simulink model "Diagram"  (R2015b)
settings: Solver=VariableStepAuto  StartTime=0.0  StopTime=0.15  RelTol=1e-3
undefined symbols (not defined in the file): K2, L2, sysog
libraries: simulink x1
settings Model: Creator=zap  LastModifiedBy=zap

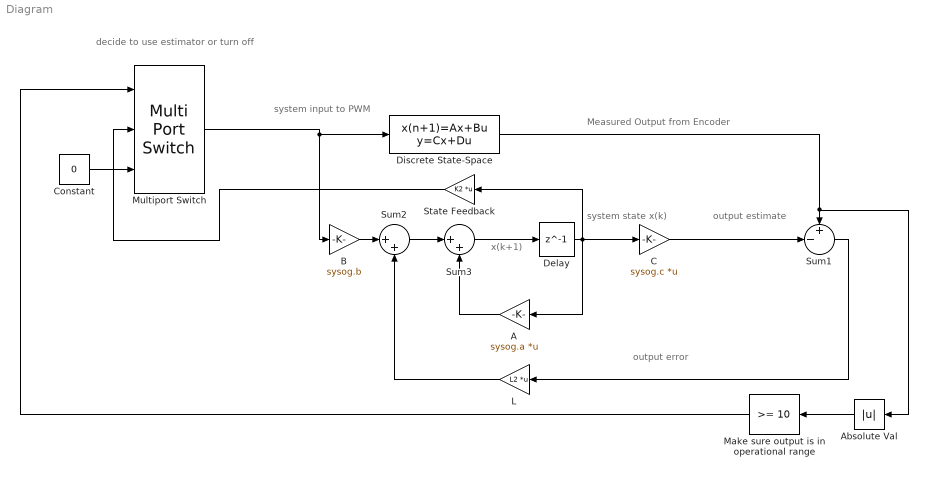
== system Diagram ==
  note: decide to use estimator or turn off
  note: system input to PWM
  note: x(k+1)
  note: system
      | state x(k)
  note: output error
  note: Measured Output from Encoder
  note: output estimate
  A : Gain  Gain=sysog.a  Multiplication=Matrix(K*u)
  Absolute Val : Abs
  B : Gain  Gain=sysog.b
  C : Gain  Gain=sysog.c  Multiplication=Matrix(K*u)
  Constant : Constant  Value=0
  Delay : Delay  DelayLength=1  InitialCondition=0
  Discrete State-Space : DiscreteStateSpace  A=sysog.a  B=sysog.b  C=sysog.c  D=sysog.d  SampleTime=10^-4
  L : Gain  Gain=L2  Multiplication=Matrix(K*u)
  Make sure output is in operational range : simulink/Logic and Bit Operations/Compare To Constant  relop=>=  const=10  OutDataTypeStr=boolean
  Multiport Switch : MultiPortSwitch  Inputs=2
  State Feedback : Gain  Gain=K2  Multiplication=Matrix(K*u)
  Sum1 : Sum  Inputs=+-|
  Sum2 : Sum  Inputs=|++
  Sum3 : Sum  Inputs=|++
  wires:
  Discrete State-Space/1 -> Absolute Val/1, Sum1/1
  Multiport Switch/1 -> B/1, Discrete State-Space/1
  B/1 -> Sum2/1
  Sum2/1 -> Sum3/1
  Sum3/1 -> Delay/1
  A/1 -> Sum3/2
  Delay/1 -> State Feedback/1, C/1, A/1
  C/1 -> Sum1/2
  Sum1/1 -> L/1
  L/1 -> Sum2/2
  State Feedback/1 -> Multiport Switch/2
  Absolute Val/1 -> Make sure output is in operational range/1
  Constant/1 -> Multiport Switch/3
  Make sure output is in operational range/1 -> Multiport Switch/1
